simulink model "Fig_9_10__"  (R2024a)
settings: Solver=VariableStepAuto  StartTime=0.0  StopTime=1  RelTol=1e-3
libraries: spsSeriesRLCBranchLib x8, spsThreePhaseVIMeasurementLib x4, spsVoltageMeasurementLib x3, slpidlib x3, spsUniversalBridgeLib x2, spsDiodeLib x2, spsIGBTDiodeLib x2, spsPWMGeneratorDCDCLib x2, spsabctodq0Lib x2, spsCurrentMeasurementLib x2, spsThreePhaseSeriesRLCBranchLib x2, spsThreePhaseSeriesRLCLoadLib x2
settings Model: Creator=MS  LastModifiedBy=Dileep Uppara

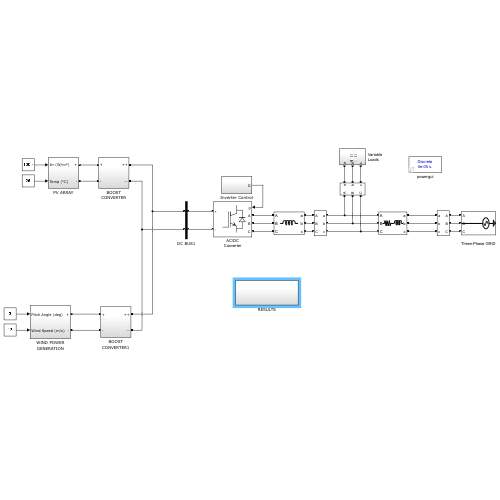
[thumbnail: Simulink's stored preview of the top-level diagram]
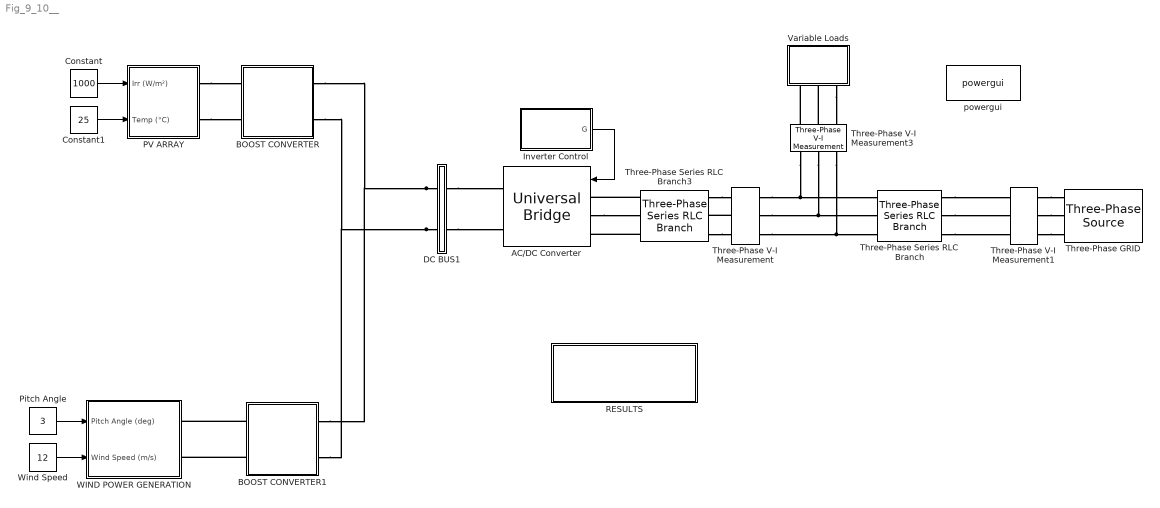
== system Fig_9_10__ ==
  " Three-Phase GRID" : spsThreePhaseSourceLib/Three-Phase Source  InternalConnection=Yg  VoltagePhases=off  Voltage=400  PhaseAngle=0  Voltage_phases=[25e3 25e3 25e3]/sqrt(3)  PhaseAngles_phases=[0 -120 +120]  Frequency=50  NonIdealSource=on  SpecifyImpedance=off  Resistance=0  Inductance=0  ShortCircuitLevel=100e6  BaseVoltage=0  XRratio=7  BusType=swing  Pref=0  Qref=0  Prefabc=[10e3, 10e3, 10e3]  Qrefabc=[0, 0, 0]  Qmin=-inf  Qmax=inf
  AC/DC Converter : spsUniversalBridgeLib/Universal Bridge  Arms=3  SnubberResistance=1e5  SnubberCapacitance=inf  Device=IGBT / Diodes  Ron=1e-3  Lon=0  ForwardVoltages="[  0  0  ]"  ForwardVoltage=0  GTOparameters=[ 10e-6 , 20e-6 ]  IGBTparameters=[ 1e-6 , 2e-6 ]  Measurements=None  Measurements_2=None  converterType=Rectifier
  BOOST CONVERTER : Subsystem
  BOOST CONVERTER1 : Subsystem
  Constant : Constant  Value=1000  SampleTime=50e-6
  Constant1 : Constant  Value=25  SampleTime=50e-6
  DC BUS1 : Subsystem
  Inverter Control : Subsystem
  PV ARRAY : Subsystem
  "Pitch Angle " : Constant  Value=3  SampleTime=50e-6
  RESULTS : Subsystem
  Three-Phase Series RLC Branch : spsThreePhaseSeriesRLCBranchLib/Three-Phase Series RLC Branch  LConnTagsString=A|B|C  RConnTagsString=A|B|C  BranchType=RL  Resistance=2.088  Inductance=0.01e-3  Capacitance=1e-6  Measurements=None
  Three-Phase Series RLC Branch3 : spsThreePhaseSeriesRLCBranchLib/Three-Phase Series RLC Branch  LConnTagsString=A|B|C  RConnTagsString=A|B|C  BranchType=L  Resistance=3  Inductance=20e-3  Capacitance=1e-6  Measurements=None
  Three-Phase V-I Measurement : spsThreePhaseVIMeasurementLib/Three-Phase V-I Measurement  VoltageMeasurement=phase-to-ground  SetLabelV=on  LabelV=Viabc  Vpu=off  VpuLL=off  CurrentMeasurement=yes  SetLabelI=on  LabelI=Iiabc  Ipu=off  Pbase=100e6  Vbase=500e3  OutputType=Complex  PhasorSimulation=off  PSBequivalent=0
  Three-Phase V-I Measurement1 : spsThreePhaseVIMeasurementLib/Three-Phase V-I Measurement  VoltageMeasurement=phase-to-ground  SetLabelV=on  LabelV=Vgabc  Vpu=off  VpuLL=off  CurrentMeasurement=yes  SetLabelI=on  LabelI=Igabc  Ipu=off  Pbase=100e6  Vbase=500e3  OutputType=Complex  PhasorSimulation=off  PSBequivalent=0
  Three-Phase V-I Measurement3 : spsThreePhaseVIMeasurementLib/Three-Phase V-I Measurement  VoltageMeasurement=phase-to-ground  SetLabelV=on  LabelV=Vlabc  Vpu=off  VpuLL=off  CurrentMeasurement=yes  SetLabelI=on  LabelI=Ilabc  Ipu=off  Pbase=100e6  Vbase=500e3  OutputType=Complex  PhasorSimulation=off  PSBequivalent=0
  Variable Loads : Subsystem
  WIND POWER GENERATION : Subsystem
  Wind Speed : Constant  Value=12  SampleTime=50e-6
  powergui : sps_lib/powergui  Priority=1  SimulationMode=Discrete  SampleTime=50e-6  frequency=60  Iterations=50  frequencyindice=0  Pbase=100e6  ErrMax=1e-4  UnitsV=kV  UnitsW=MW  buscounter=0  FunctionMessages=off  echomessages=off  EnableUseOfTLC=off  CurrentSourceSwitches=off  DisableSnubberDevices=off  DisableRonSwitches=off  DisableVfSwitches=off  DisplayEquations=off  AutomaticDiscreteSolvers=off  SolverType=Tustin/Backward Euler (TBE)  Interpol=off  ExternalGateDelay=off  methode=off  Ts=100  x0status=blocks  SPID=on  SwTol=0  HookPort=off  NonlinearTolerance=1e-4  nMaxIteration=100  ContinueOnMaxIteration=off  RestoreLinks=warning  ResistiveCurrentMeasurement=off  Frange=[0:2:500]  Ylog=off  Xlog=on  ShowGrid=off  save=off  variable=ZData  structure=0  ZoomFFT=off  StartTime=0.0  cycles=1  DisplayStyle=1  fundamental=60  FreqAxis=off  MaxFrequency=1000  frequencyindicesteady=1  RmsSteady=1  display=off
  wires:
  Inverter Control/1(G) -> AC/DC Converter/1
  Constant/1 -> PV ARRAY/1(Irr (W/m²))
  Constant1/1 -> PV ARRAY/2(Temp (°C))
  Wind Speed/1 -> WIND POWER GENERATION/2(Wind Speed (m/s))
  "Pitch Angle "/1 -> WIND POWER GENERATION/1(Pitch Angle (deg))
  connections:
  Three-Phase Series RLC Branch3/LConn1 -- AC/DC Converter/LConn1
  AC/DC Converter/LConn2 -- Three-Phase Series RLC Branch3/LConn2
  Three-Phase Series RLC Branch3/LConn3 -- AC/DC Converter/LConn3
  Three-Phase Series RLC Branch3/RConn1 -- Three-Phase V-I Measurement/LConn1
  Three-Phase V-I Measurement/LConn2 -- Three-Phase Series RLC Branch3/RConn2
  Three-Phase Series RLC Branch3/RConn3 -- Three-Phase V-I Measurement/LConn3
  DC BUS1/RConn2 -- AC/DC Converter/RConn2
  DC BUS1/RConn1 -- AC/DC Converter/RConn1
  Three-Phase V-I Measurement3/LConn1 -- Three-Phase Series RLC Branch/LConn1 -- Three-Phase V-I Measurement/RConn1
  Three-Phase V-I Measurement3/LConn3 -- Three-Phase Series RLC Branch/LConn3 -- Three-Phase V-I Measurement/RConn3
  Three-Phase V-I Measurement3/LConn2 -- Three-Phase V-I Measurement/RConn2 -- Three-Phase Series RLC Branch/LConn2
  Three-Phase V-I Measurement1/LConn3 -- " Three-Phase GRID"/RConn3
  Three-Phase Series RLC Branch/RConn1 -- Three-Phase V-I Measurement1/RConn1
  Three-Phase V-I Measurement1/LConn1 -- " Three-Phase GRID"/RConn1
  Three-Phase Series RLC Branch/RConn2 -- Three-Phase V-I Measurement1/RConn2
  Three-Phase V-I Measurement1/LConn2 -- " Three-Phase GRID"/RConn2
  Three-Phase Series RLC Branch/RConn3 -- Three-Phase V-I Measurement1/RConn3
  DC BUS1/LConn2 -- BOOST CONVERTER1/RConn2 -- BOOST CONVERTER/RConn2
  DC BUS1/LConn1 -- BOOST CONVERTER1/RConn1 -- BOOST CONVERTER/RConn1
  Three-Phase V-I Measurement3/RConn2 -- Variable Loads/LConn2
  Three-Phase V-I Measurement3/RConn1 -- Variable Loads/LConn1
  Variable Loads/LConn3 -- Three-Phase V-I Measurement3/RConn3
  PV ARRAY/RConn1 -- BOOST CONVERTER/LConn1
  BOOST CONVERTER1/LConn1 -- WIND POWER GENERATION/RConn1
  BOOST CONVERTER1/LConn2 -- WIND POWER GENERATION/RConn2
  PV ARRAY/RConn2 -- BOOST CONVERTER/LConn2

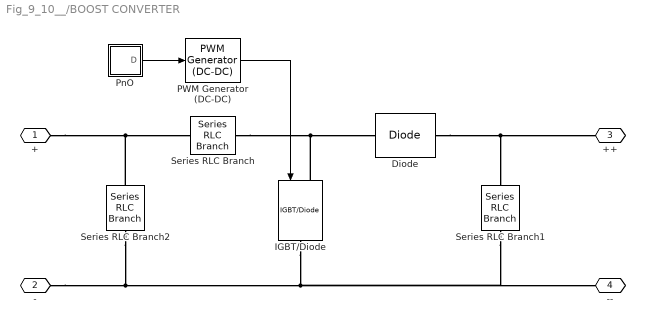
== system Fig_9_10__/BOOST CONVERTER ==
  Diode : spsDiodeLib/Diode  Ron=0.001  Lon=0  Vf=0.8  IC=0  UseSnubber=0  Rs=500  Cs=250e-9  Measurements=off
  IGBT/Diode : spsIGBTDiodeLib/IGBT//Diode  Ron=1e-3  Rs=1e5  Cs=inf  Measurements=off
  PWM Generator (DC-DC) : spsPWMGeneratorDCDCLib/PWM Generator (DC-DC)  Fsw=15e3  Ts=50e-6
  PnO : Subsystem
  Series RLC Branch : spsSeriesRLCBranchLib/Series RLC Branch  LConnTagsString=__new0  RConnTagsString=__new0  BranchType=L  Resistance=0.01  Inductance=0.009e-3  SetiL0=off  InitialCurrent=0  Capacitance=1e-6  Setx0=off  InitialVoltage=0  Measurements=None
  Series RLC Branch1 : spsSeriesRLCBranchLib/Series RLC Branch  LConnTagsString=__new0  RConnTagsString=__new0  BranchType=C  Resistance=0.01  Inductance=0.5e-3  SetiL0=off  InitialCurrent=0  Capacitance=880e-6  Setx0=off  InitialVoltage=0  Measurements=None
  Series RLC Branch2 : spsSeriesRLCBranchLib/Series RLC Branch  LConnTagsString=__new0  RConnTagsString=__new0  BranchType=C  Resistance=0.01  Inductance=0.5e-3  SetiL0=off  InitialCurrent=0  Capacitance=880e-6  Setx0=off  InitialVoltage=0  Measurements=None
  + : PMIOPort  Side=Left
  - : PMIOPort  Port=2  Side=Left
  ++ : PMIOPort  Port=3  Side=Right
  -- : PMIOPort  Port=4  Side=Right
  wires:
  PWM Generator (DC-DC)/1 -> IGBT/Diode/1
  PnO/1(D) -> PWM Generator (DC-DC)/1
  connections:
  Series RLC Branch/RConn1 -- Diode/LConn1 -- IGBT/Diode/LConn1
  +/RConn1 -- Series RLC Branch2/LConn1 -- Series RLC Branch/LConn1
  Series RLC Branch2/RConn1 -- -/RConn1 -- Series RLC Branch1/RConn1 -- --/RConn1 -- IGBT/Diode/RConn1
  Diode/RConn1 -- ++/RConn1 -- Series RLC Branch1/LConn1

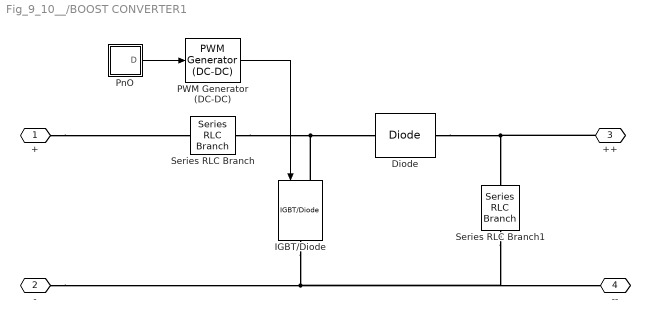
== system Fig_9_10__/BOOST CONVERTER1 ==
  Diode : spsDiodeLib/Diode  Ron=0.001  Lon=0  Vf=0.8  IC=0  UseSnubber=0  Rs=500  Cs=250e-9  Measurements=off
  IGBT/Diode : spsIGBTDiodeLib/IGBT//Diode  Ron=1e-3  Rs=1e5  Cs=inf  Measurements=off
  PWM Generator (DC-DC) : spsPWMGeneratorDCDCLib/PWM Generator (DC-DC)  Fsw=15e3  Ts=50e-6
  PnO : Subsystem
  Series RLC Branch : spsSeriesRLCBranchLib/Series RLC Branch  LConnTagsString=__new0  RConnTagsString=__new0  BranchType=RL  Resistance=1.524  Inductance=0.1e-3  SetiL0=off  InitialCurrent=0  Capacitance=1e-6  Setx0=off  InitialVoltage=0  Measurements=None
  Series RLC Branch1 : spsSeriesRLCBranchLib/Series RLC Branch  LConnTagsString=__new0  RConnTagsString=__new0  BranchType=C  Resistance=0.01  Inductance=0.5e-3  SetiL0=off  InitialCurrent=0  Capacitance=880e-6  Setx0=off  InitialVoltage=0  Measurements=None
  + : PMIOPort  Side=Left
  - : PMIOPort  Port=2  Side=Left
  ++ : PMIOPort  Port=3  Side=Right
  -- : PMIOPort  Port=4  Side=Right
  wires:
  PWM Generator (DC-DC)/1 -> IGBT/Diode/1
  PnO/1(D) -> PWM Generator (DC-DC)/1
  connections:
  Series RLC Branch/RConn1 -- Diode/LConn1 -- IGBT/Diode/LConn1
  Diode/RConn1 -- Series RLC Branch1/LConn1 -- ++/RConn1
  +/RConn1 -- Series RLC Branch/LConn1
  -/RConn1 -- Series RLC Branch1/RConn1 -- --/RConn1 -- IGBT/Diode/RConn1

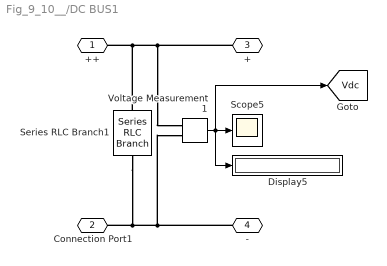
== system Fig_9_10__/DC BUS1 ==
  Display5 : Display
  Scope5 : Scope
  Series RLC Branch1 : spsSeriesRLCBranchLib/Series RLC Branch  LConnTagsString=__new0  RConnTagsString=__new0  BranchType=C  Resistance=0.01  Inductance=0.5e-3  SetiL0=off  InitialCurrent=0  Capacitance=10000e-6  Setx0=off  InitialVoltage=0  Measurements=None
  Voltage Measurement1 : spsVoltageMeasurementLib/Voltage Measurement  PhasorSimulation=off  OutputType=Complex  PSBequivalent=0
  ++ : PMIOPort  Side=Left
  Connection Port1 : PMIOPort  Port=2  Side=Left
  + : PMIOPort  Port=3  Side=Right
  - : PMIOPort  Port=4  Side=Right
  tag scope: Vdc=global
  wires:
  Voltage Measurement1/1 -> [Vdc], Display5/1, Scope5/1
  connections:
  -/RConn1 -- Voltage Measurement1/LConn2 -- Series RLC Branch1/RConn1 -- Connection Port1/RConn1
  +/RConn1 -- Series RLC Branch1/LConn1 -- ++/RConn1 -- Voltage Measurement1/LConn1

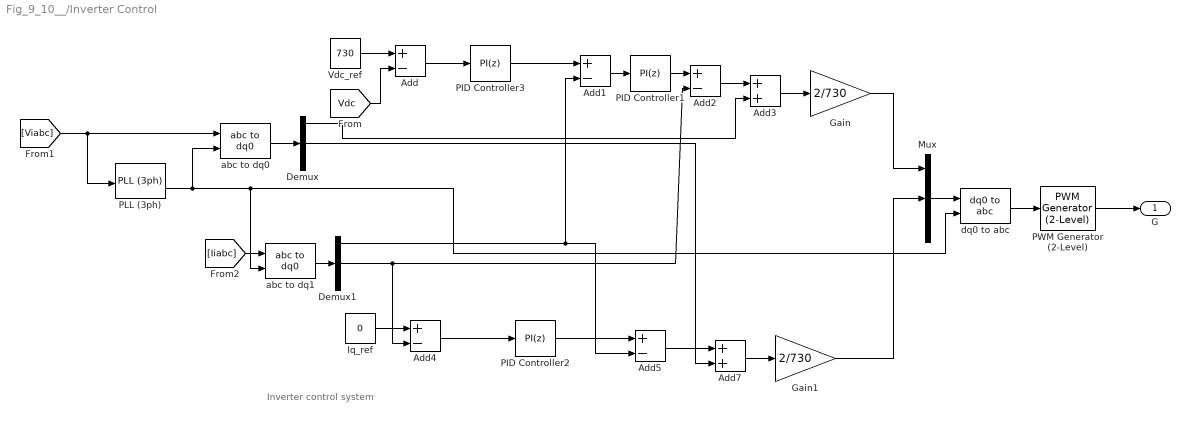
== system Fig_9_10__/Inverter Control ==
  note: Inverter control system
  Add{,1..2,4..5} (5 alike) : Sum  Inputs=+-
  Add3 : Sum
  Add7 : Sum
  Demux : Demux  Outputs=3
  Demux1 : Demux  Outputs=3
  Gain : Gain  Gain=2/730
  Gain1 : Gain  Gain=2/730
  Iq_ref : Constant  Value=0
  Mux : Mux  Inputs=3
  PID Controller1 : slpidlib/PID Controller  Controller=PI  Form=Parallel  TimeDomain=Discrete-time  UseExternalTs=off  SampleTime=-1  IntegratorMethod=Forward Euler  FilterMethod=Forward Euler  ControllerParametersSource=internal  P=0.5  I=200  UseKiTs=off  D=0  UseExternalDerivativeSource=off  N=100  UseFilter=on  TunerSelectOption=Transfer Function Based (PID Tuner App)  InitialConditionSource=internal  InitialConditionForIntegrator=0  InitialConditionForFilter=0  DifferentiatorICPrevScaledInput=0  ExternalReset=none  TrackingMode=off  Kt=1  LimitOutput=off  SatLimitsSource=internal  UpperSaturationLimit=inf  LowerSaturationLimit=-inf  LinearizeAsGain=on  AntiWindupMode=none  Kb=1  LimitIntegrator=off  UpperIntegratorSaturationLimit=inf  LowerIntegratorSaturationLimit=-inf  POutMin=[]  POutMax=[]  IOutMin=[]  IOutMax=[]  DOutMin=[]  DOutMax=[]  NOutMin=[]  NOutMax=[]  SumOutMin=[]  SumOutMax=[]  SaturationOutMin=[]  SaturationOutMax=[]  PParamMin=[]  PParamMax=[]  IParamMin=[]  IParamMax=[]  DParamMin=[]  DParamMax=[]  NParamMin=[]  NParamMax=[]  KbParamMin=[]  KbParamMax=[]  KtParamMin=[]  KtParamMax=[]  KbOutMin=[]  KbOutMax=[]  KtOutMin=[]  KtOutMax=[]  IntegratorOutMin=[]  IntegratorOutMax=[]  FilterOutMin=[]  FilterOutMax=[]  SumI1OutMin=[]  SumI1OutMax=[]  SumI2OutMin=[]  SumI2OutMax=[]  SumI3OutMin=[]  SumI3OutMax=[]  SumI4OutMin=[]  SumI4OutMax=[]  SumDOutMin=[]  SumDOutMax=[]  DifferentiatorOutMin=[]  DifferentiatorOutMax=[]  FilterDiffOutCoefMin=[]  FilterDiffOutCoefMax=[]  ReciprocalOutMin=[]  ReciprocalOutMax=[]  SumDenOutMin=[]  SumDenOutMax=[]  SumNumOutMin=[]  SumNumOutMax=[]  DivideOutMin=[]  DivideOutMax=[]  UdiffTsProdOutMin=[]  UdiffTsProdOutMax=[]  NTsProdOutMin=[]  NTsProdOutMax=[]  UintegralTsProdOutMin=[]  UintegralTsProdOutMax=[]  UngainTsProdOutMin=[]  UngainTsProdOutMax=[]  ClampingZeroOutDataTypeStr=Inherit: Inherit via back propagation  ClampingZeroOutMin=[]  ClampingZeroOutMax=[]  FilterDenConstantOutDataTypeStr=Inherit: Inherit via back propagation  FilterDenConstantOutMin=[]  FilterDenConstantOutMax=[]  PCopyOutDataTypeStr=Inherit: Inherit via back propagation  PCopyOutMin=[]  PCopyOutMax=[]  NCopyOutDataTypeStr=Inherit: Inherit via back propagation  NCopyOutMin=[]  NCopyOutMax=[]  IntegratorContinuousStateAttributes=''  IntegratorStateMustResolveToSignalObject=off  IntegratorRTWStateStorageClass=Auto  FilterContinuousStateAttributes=''  FilterStateMustResolveToSignalObject=off  FilterRTWStateStorageClass=Auto  ParallelPVariant=InternalParameters  IdealPVariant=Disabled  IVariant=InternalParameters  DVariant=Disabled  IntegratorVariant=Discrete  SatVariant=Disabled  AWVariant=Passthrough  PCopyVariant=Disabled  TRVariant=Disabled  FdbkBlocksVariant=Forward  IdealPFdbkVariant=Disabled  SatFdbkVariant=Disabled  DerivativeFilterVariant=Disabled  NVariant=Disabled  NCopyVariant=Disabled_SignalSpec  FilterICVariant=Disabled  IntegratorICVariant=InternalICs  ExternalResetVariant=Disabled  TRSumVariant=Passthrough  SumFdbkVariant=Disabled  SumVariant=Sum_PI  TsampFilterVariant=InternalTs  TsampNgainVariant=Passthrough  TsampIntegralVariant=Disabled_SignalSpec  ExternalSaturationOutDataTypeStr=Inherit: Same as second input  DerivativeSourceVariant=Disabled
  PID Controller2 : slpidlib/PID Controller  Controller=PI  Form=Parallel  TimeDomain=Discrete-time  UseExternalTs=off  SampleTime=-1  IntegratorMethod=Forward Euler  FilterMethod=Forward Euler  ControllerParametersSource=internal  P=0.5  I=200  UseKiTs=off  D=0  UseExternalDerivativeSource=off  N=100  UseFilter=on  TunerSelectOption=Transfer Function Based (PID Tuner App)  InitialConditionSource=internal  InitialConditionForIntegrator=0  InitialConditionForFilter=0  DifferentiatorICPrevScaledInput=0  ExternalReset=none  TrackingMode=off  Kt=1  LimitOutput=off  SatLimitsSource=internal  UpperSaturationLimit=inf  LowerSaturationLimit=-inf  LinearizeAsGain=on  AntiWindupMode=none  Kb=1  LimitIntegrator=off  UpperIntegratorSaturationLimit=inf  LowerIntegratorSaturationLimit=-inf  POutMin=[]  POutMax=[]  IOutMin=[]  IOutMax=[]  DOutMin=[]  DOutMax=[]  NOutMin=[]  NOutMax=[]  SumOutMin=[]  SumOutMax=[]  SaturationOutMin=[]  SaturationOutMax=[]  PParamMin=[]  PParamMax=[]  IParamMin=[]  IParamMax=[]  DParamMin=[]  DParamMax=[]  NParamMin=[]  NParamMax=[]  KbParamMin=[]  KbParamMax=[]  KtParamMin=[]  KtParamMax=[]  KbOutMin=[]  KbOutMax=[]  KtOutMin=[]  KtOutMax=[]  IntegratorOutMin=[]  IntegratorOutMax=[]  FilterOutMin=[]  FilterOutMax=[]  SumI1OutMin=[]  SumI1OutMax=[]  SumI2OutMin=[]  SumI2OutMax=[]  SumI3OutMin=[]  SumI3OutMax=[]  SumI4OutMin=[]  SumI4OutMax=[]  SumDOutMin=[]  SumDOutMax=[]  DifferentiatorOutMin=[]  DifferentiatorOutMax=[]  FilterDiffOutCoefMin=[]  FilterDiffOutCoefMax=[]  ReciprocalOutMin=[]  ReciprocalOutMax=[]  SumDenOutMin=[]  SumDenOutMax=[]  SumNumOutMin=[]  SumNumOutMax=[]  DivideOutMin=[]  DivideOutMax=[]  UdiffTsProdOutMin=[]  UdiffTsProdOutMax=[]  NTsProdOutMin=[]  NTsProdOutMax=[]  UintegralTsProdOutMin=[]  UintegralTsProdOutMax=[]  UngainTsProdOutMin=[]  UngainTsProdOutMax=[]  ClampingZeroOutDataTypeStr=Inherit: Inherit via back propagation  ClampingZeroOutMin=[]  ClampingZeroOutMax=[]  FilterDenConstantOutDataTypeStr=Inherit: Inherit via back propagation  FilterDenConstantOutMin=[]  FilterDenConstantOutMax=[]  PCopyOutDataTypeStr=Inherit: Inherit via back propagation  PCopyOutMin=[]  PCopyOutMax=[]  NCopyOutDataTypeStr=Inherit: Inherit via back propagation  NCopyOutMin=[]  NCopyOutMax=[]  IntegratorContinuousStateAttributes=''  IntegratorStateMustResolveToSignalObject=off  IntegratorRTWStateStorageClass=Auto  FilterContinuousStateAttributes=''  FilterStateMustResolveToSignalObject=off  FilterRTWStateStorageClass=Auto  ParallelPVariant=InternalParameters  IdealPVariant=Disabled  IVariant=InternalParameters  DVariant=Disabled  IntegratorVariant=Discrete  SatVariant=Disabled  AWVariant=Passthrough  PCopyVariant=Disabled  TRVariant=Disabled  FdbkBlocksVariant=Forward  IdealPFdbkVariant=Disabled  SatFdbkVariant=Disabled  DerivativeFilterVariant=Disabled  NVariant=Disabled  NCopyVariant=Disabled_SignalSpec  FilterICVariant=Disabled  IntegratorICVariant=InternalICs  ExternalResetVariant=Disabled  TRSumVariant=Passthrough  SumFdbkVariant=Disabled  SumVariant=Sum_PI  TsampFilterVariant=InternalTs  TsampNgainVariant=Passthrough  TsampIntegralVariant=Disabled_SignalSpec  ExternalSaturationOutDataTypeStr=Inherit: Same as second input  DerivativeSourceVariant=Disabled
  PID Controller3 : slpidlib/PID Controller  Controller=PI  Form=Parallel  TimeDomain=Discrete-time  UseExternalTs=off  SampleTime=-1  IntegratorMethod=Forward Euler  FilterMethod=Forward Euler  ControllerParametersSource=internal  P=1  I=500  UseKiTs=off  D=0  UseExternalDerivativeSource=off  N=100  UseFilter=on  TunerSelectOption=Transfer Function Based (PID Tuner App)  InitialConditionSource=internal  InitialConditionForIntegrator=0  InitialConditionForFilter=0  DifferentiatorICPrevScaledInput=0  ExternalReset=none  TrackingMode=off  Kt=1  LimitOutput=off  SatLimitsSource=internal  UpperSaturationLimit=inf  LowerSaturationLimit=-inf  LinearizeAsGain=on  AntiWindupMode=none  Kb=1  LimitIntegrator=off  UpperIntegratorSaturationLimit=inf  LowerIntegratorSaturationLimit=-inf  POutMin=[]  POutMax=[]  IOutMin=[]  IOutMax=[]  DOutMin=[]  DOutMax=[]  NOutMin=[]  NOutMax=[]  SumOutMin=[]  SumOutMax=[]  SaturationOutMin=[]  SaturationOutMax=[]  PParamMin=[]  PParamMax=[]  IParamMin=[]  IParamMax=[]  DParamMin=[]  DParamMax=[]  NParamMin=[]  NParamMax=[]  KbParamMin=[]  KbParamMax=[]  KtParamMin=[]  KtParamMax=[]  KbOutMin=[]  KbOutMax=[]  KtOutMin=[]  KtOutMax=[]  IntegratorOutMin=[]  IntegratorOutMax=[]  FilterOutMin=[]  FilterOutMax=[]  SumI1OutMin=[]  SumI1OutMax=[]  SumI2OutMin=[]  SumI2OutMax=[]  SumI3OutMin=[]  SumI3OutMax=[]  SumI4OutMin=[]  SumI4OutMax=[]  SumDOutMin=[]  SumDOutMax=[]  DifferentiatorOutMin=[]  DifferentiatorOutMax=[]  FilterDiffOutCoefMin=[]  FilterDiffOutCoefMax=[]  ReciprocalOutMin=[]  ReciprocalOutMax=[]  SumDenOutMin=[]  SumDenOutMax=[]  SumNumOutMin=[]  SumNumOutMax=[]  DivideOutMin=[]  DivideOutMax=[]  UdiffTsProdOutMin=[]  UdiffTsProdOutMax=[]  NTsProdOutMin=[]  NTsProdOutMax=[]  UintegralTsProdOutMin=[]  UintegralTsProdOutMax=[]  UngainTsProdOutMin=[]  UngainTsProdOutMax=[]  ClampingZeroOutDataTypeStr=Inherit: Inherit via back propagation  ClampingZeroOutMin=[]  ClampingZeroOutMax=[]  FilterDenConstantOutDataTypeStr=Inherit: Inherit via back propagation  FilterDenConstantOutMin=[]  FilterDenConstantOutMax=[]  PCopyOutDataTypeStr=Inherit: Inherit via back propagation  PCopyOutMin=[]  PCopyOutMax=[]  NCopyOutDataTypeStr=Inherit: Inherit via back propagation  NCopyOutMin=[]  NCopyOutMax=[]  IntegratorContinuousStateAttributes=''  IntegratorStateMustResolveToSignalObject=off  IntegratorRTWStateStorageClass=Auto  FilterContinuousStateAttributes=''  FilterStateMustResolveToSignalObject=off  FilterRTWStateStorageClass=Auto  ParallelPVariant=InternalParameters  IdealPVariant=Disabled  IVariant=InternalParameters  DVariant=Disabled  IntegratorVariant=Discrete  SatVariant=Disabled  AWVariant=Passthrough  PCopyVariant=Disabled  TRVariant=Disabled  FdbkBlocksVariant=Forward  IdealPFdbkVariant=Disabled  SatFdbkVariant=Disabled  DerivativeFilterVariant=Disabled  NVariant=Disabled  NCopyVariant=Disabled_SignalSpec  FilterICVariant=Disabled  IntegratorICVariant=InternalICs  ExternalResetVariant=Disabled  TRSumVariant=Passthrough  SumFdbkVariant=Disabled  SumVariant=Sum_PI  TsampFilterVariant=InternalTs  TsampNgainVariant=Passthrough  TsampIntegralVariant=Disabled_SignalSpec  ExternalSaturationOutDataTypeStr=Inherit: Same as second input  DerivativeSourceVariant=Disabled
  PLL (3ph) : spsPLL3phLib/PLL (3ph)  Fmin=45  Par_Init=[0, 50]  ParK=[180, 3200, 1]  TcD=1e-4  MaxRateChangeFreq=12  FilterCutOffFreq=25  Ts=50e-6  AGC=on
  PWM Generator (2-Level) : spsPWMGenerator2LevelLib/PWM Generator (2-Level)  ModulatorType=Three-phase bridge (6 pulses)  ModulatorMode=Unsynchronized  Fc=20e3  Pc=90  nF=27  MinMax="[ -1  1 ]"  SamplingTechnique=Natural  ModulatingSignals=off  m=0.8  Freq=50  Phase=0  Ts=50e-6  ShowCarrierOutport=off
  Vdc_ref : Constant  Value=730
  abc to dq0 : spsabctodq0Lib/abc to dq0  Alignment=90 degrees behind phase A axis
  abc to dq1 : spsabctodq0Lib/abc to dq0  Alignment=90 degrees behind phase A axis
  dq0 to abc : spsdq0toabcLib/dq0 to abc  Alignment=90 degrees behind phase A axis
  G : Outport
  wires:
  Vdc_ref/1 -> Add/1
  [Vdc] -> Add/2
  Add1/1 -> PID Controller1/1
  PID Controller1/1 -> Add2/1
  Add2/1 -> Add3/1
  Add3/1 -> Gain/1
  abc to dq0/1 -> Demux/1
  [Viabc] -> PLL (3ph)/1, abc to dq0/1
  PLL (3ph)/2 -> dq0 to abc/2, abc to dq1/2, abc to dq0/2
  [Iiabc] -> abc to dq1/1
  abc to dq1/1 -> Demux1/1
  Add5/1 -> Add7/1
  PID Controller2/1 -> Add5/1
  Add4/1 -> PID Controller2/1
  Demux1/2 -> Add4/2, Add2/2
  Iq_ref/1 -> Add4/1
  Demux/1 -> Add3/2
  Demux1/1 -> Add5/2, Add1/2
  Add7/1 -> Gain1/1
  Demux/2 -> Add7/2
  Gain/1 -> Mux/1
  Mux/1 -> dq0 to abc/1
  Gain1/1 -> Mux/2
  dq0 to abc/1 -> PWM Generator (2-Level)/1
  PWM Generator (2-Level)/1 -> G/1
  PID Controller3/1 -> Add1/1
  Add/1 -> PID Controller3/1

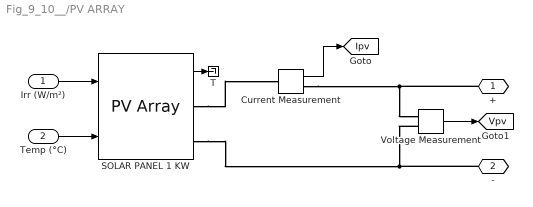
== system Fig_9_10__/PV ARRAY ==
  Irr (W/m²) : Inport
  Temp (°C) : Inport  Port=2
  Current Measurement : spsCurrentMeasurementLib/Current Measurement  PhasorSimulation=off  OutputType=Complex  PSBequivalent=0
  SOLAR PANEL 1 KW : spsPVArrayLib/PV Array  Npar=44  Nser=18  PlotType=array @ 1000 W/m2 & specified temperatures  S_vec="[ 1000  500  100 ]"  Temp_C_vec="[ 45 25  ]"  ModuleName=User-defined  PlotWhenSelected=off  Pm=214.6493  Ncell=60  Voc=36.3  Isc=7.84  Vm=29  Im=7.4017  beta_Voc_pc=-0.36099  alpha_Isc_pc=0.102  beta_Voc=-0.13104  alpha_Isc=0.0079968  IL=7.9095  I0=2.9374e-10  nI=0.98114  Rsh=294.0158  Rs=0.39142  RobustModel=off  RobustCellTemperature=313.3991  BAL=on  Tc=1e-6  Tfilter=5e-5
  T : Terminator
  Voltage Measurement : spsVoltageMeasurementLib/Voltage Measurement  PhasorSimulation=off  OutputType=Complex  PSBequivalent=0
  + : PMIOPort  Side=Right
  - : PMIOPort  Port=2  Side=Right
  tag scope: Ipv=global, Vpv=global
  wires:
  Voltage Measurement/1 -> [Vpv]
  Current Measurement/1 -> [Ipv]
  SOLAR PANEL 1 KW/1 -> T/1
  Irr (W/m²)/1 -> SOLAR PANEL 1 KW/1
  Temp (°C)/1 -> SOLAR PANEL 1 KW/2
  connections:
  Current Measurement/RConn1 -- +/RConn1 -- Voltage Measurement/LConn1
  Voltage Measurement/LConn2 -- -/RConn1 -- SOLAR PANEL 1 KW/RConn2
  SOLAR PANEL 1 KW/RConn1 -- Current Measurement/LConn1

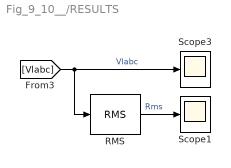
== system Fig_9_10__/RESULTS ==
  RMS : spsRMSLib/RMS  TrueRMS=on  Freq=50  RMSInit=0  Ts=50e-6
  Scope1 : Scope
  Scope3 : Scope
  wires:
  RMS/1 -> Scope1/1  "Rms"
  [Vlabc] -> RMS/1, Scope3/1  "Vlabc"

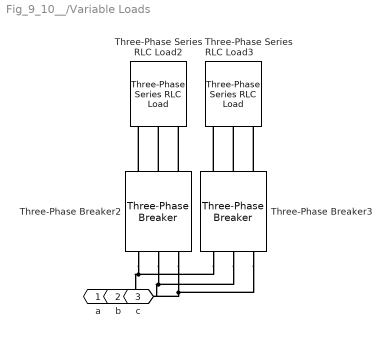
== system Fig_9_10__/Variable Loads ==
  Three-Phase Series RLC Load2 : spsThreePhaseSeriesRLCLoadLib/Three-Phase Series RLC Load  LConnTagsString=A|B|C  Configuration=Y (grounded)  NominalVoltage=400  Vabc=[1e3 1e3 1e3]  Vabcp=[1e3 1e3 1e3]  NominalFrequency=50  UnbalancedPower=off  ActivePower=20e3  InductivePower=0  CapacitivePower=0  Pabc=[10e3 9e3 11e3]  QLabc=[100 90 110]  QCabc=[100 90 110]  Pabcp=[10e3 9e3 11e3]  QLabcp=[100 90 110]  QCabcp=[100 90 110]  Measurements=None  LoadType=constant Z
  Three-Phase Series RLC Load3 : spsThreePhaseSeriesRLCLoadLib/Three-Phase Series RLC Load  LConnTagsString=A|B|C  Configuration=Y (grounded)  NominalVoltage=400  Vabc=[1e3 1e3 1e3]  Vabcp=[1e3 1e3 1e3]  NominalFrequency=50  UnbalancedPower=off  ActivePower=20e3  InductivePower=0  CapacitivePower=0  Pabc=[10e3 9e3 11e3]  QLabc=[100 90 110]  QCabc=[100 90 110]  Pabcp=[10e3 9e3 11e3]  QLabcp=[100 90 110]  QCabcp=[100 90 110]  Measurements=None  LoadType=constant Z
  Three-Phase Breaker2 : spsThreePhaseBreakerLib/Three-Phase Breaker  InitialState=open  SwitchA=on  SwitchB=on  SwitchC=on  SwitchTimes=[0.2 0.4]  External=off  BreakerResistance=0.01  SnubberResistance=1e6  SnubberCapacitance=inf  Measurements=None
  Three-Phase Breaker3 : spsThreePhaseBreakerLib/Three-Phase Breaker  InitialState=closed  SwitchA=on  SwitchB=on  SwitchC=on  SwitchTimes=[0.6 0.8]  External=off  BreakerResistance=0.01  SnubberResistance=1e6  SnubberCapacitance=inf  Measurements=None
  a : PMIOPort  Side=Left
  b : PMIOPort  Port=2  Side=Left
  c : PMIOPort  Port=3  Side=Left
  connections:
  Three-Phase Breaker2/LConn3 -- Three-Phase Series RLC Load2/LConn3
  Three-Phase Breaker3/LConn3 -- Three-Phase Series RLC Load3/LConn3
  Three-Phase Breaker2/RConn3 -- c/RConn1 -- Three-Phase Breaker3/RConn3
  Three-Phase Breaker2/RConn2 -- b/RConn1 -- Three-Phase Breaker3/RConn2
  Three-Phase Breaker3/LConn2 -- Three-Phase Series RLC Load3/LConn2
  Three-Phase Breaker2/RConn1 -- a/RConn1 -- Three-Phase Breaker3/RConn1
  Three-Phase Breaker2/LConn2 -- Three-Phase Series RLC Load2/LConn2
  Three-Phase Breaker3/LConn1 -- Three-Phase Series RLC Load3/LConn1
  Three-Phase Breaker2/LConn1 -- Three-Phase Series RLC Load2/LConn1

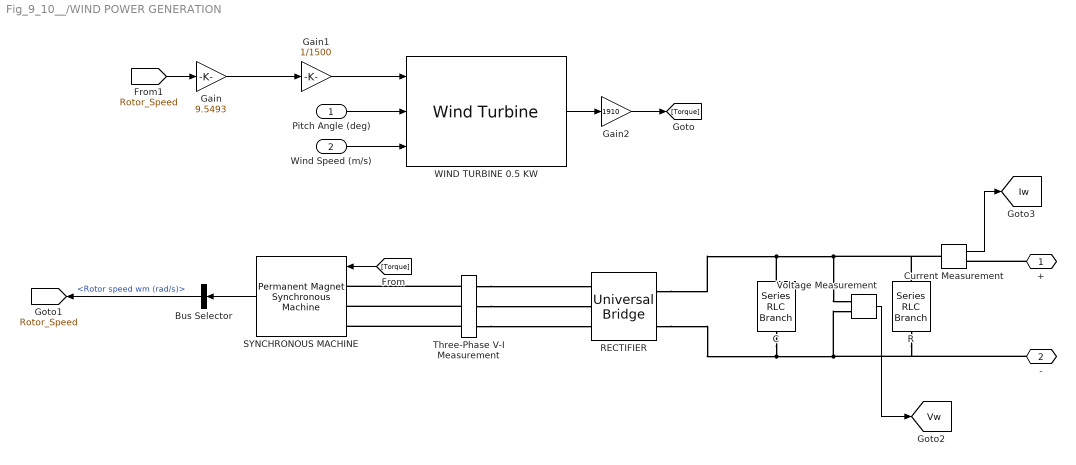
== system Fig_9_10__/WIND POWER GENERATION ==
  Pitch Angle (deg) : Inport
  Wind Speed (m/s) : Inport  Port=2
  Bus Selector : BusSelector  OutputSignals=Rotor speed wm (rad/s)
  C : spsSeriesRLCBranchLib/Series RLC Branch  LConnTagsString=__new0  RConnTagsString=__new0  BranchType=C  Resistance=20  Inductance=1e-3  SetiL0=off  InitialCurrent=0  Capacitance=1000e-6  Setx0=off  InitialVoltage=0  Measurements=None
  Current Measurement : spsCurrentMeasurementLib/Current Measurement  PhasorSimulation=off  OutputType=Complex  PSBequivalent=0
  Gain : Gain  Gain=9.5493
  Gain1 : Gain  Gain=1/1500
  Gain2 : Gain  Gain=1910
  R : spsSeriesRLCBranchLib/Series RLC Branch  LConnTagsString=__new0  RConnTagsString=__new0  BranchType=R  Resistance=15  Inductance=1e-3  SetiL0=off  InitialCurrent=0  Capacitance=10e-3  Setx0=off  InitialVoltage=0  Measurements=None
  RECTIFIER : spsUniversalBridgeLib/Universal Bridge  Arms=3  SnubberResistance=1e5  SnubberCapacitance=inf  Device=Diodes  Ron=1e-3  Lon=0  ForwardVoltages="[  0  0  ]"  ForwardVoltage=0  GTOparameters=[ 10e-6 , 20e-6 ]  IGBTparameters=[ 1e-6 , 2e-6 ]  Measurements=None  Measurements_2=None  converterType=Rectifier
  SYNCHRONOUS MACHINE : spsPermanentMagnetSynchronousMachineLib/Permanent Magnet Synchronous Machine  NbPhases=3  FluxDistribution=Sinusoidal  RotorType=Round  MechanicalLoad=Torque Tm  PresetModel=No  ShowDetailedParameters=on  MeasurementBus=off  Resistance=0.0485  Inductance=8.5e-3  dqInductances=[8.5e-3,8.5e-3]  La=0.000395  MachineConstant=Flux linkage established by magnets (V.s)  Flux=1.2  VoltageCst=870.6237  TorqueCst=7.2  Flat=120  Mechanical=[0.0027 0.0004924 4 0]  PolePairs=4  InitialConditions=[0,0, 0,0]  InitialConditions5ph=[0 0 0 0 0 0]  RefAngle=90 degrees behind phase A axis (modified Park)  IterativeDiscreteModel=Trapezoidal non iterative  TsBlock=50e-6  TsPowergui=0
  Three-Phase V-I Measurement : spsThreePhaseVIMeasurementLib/Three-Phase V-I Measurement  VoltageMeasurement=phase-to-phase  SetLabelV=on  LabelV=Vabc  Vpu=off  VpuLL=off  CurrentMeasurement=yes  SetLabelI=on  LabelI=Iabc  Ipu=off  Pbase=100e6  Vbase=500e3  OutputType=Complex  PhasorSimulation=off  PSBequivalent=0
  Voltage Measurement : spsVoltageMeasurementLib/Voltage Measurement  PhasorSimulation=off  OutputType=Complex  PSBequivalent=0
  WIND TURBINE 0.5 KW : spsWindTurbineLib/Wind Turbine  Pnom=300e3  Pelec_base=300e3/0.9  wind_base=12  P_wind_base=0.73  speed_nom=1.2  pitch_angle=0  c1_c6="[0.51763          116          0.4            5           21     0.006795]"  cp_nom=0.48  lambda_nom=8.1
  + : PMIOPort  Side=Right
  - : PMIOPort  Port=2  Side=Right
  tag scope: Iw=global, Rotor_Speed=global, Vw=global
  wires:
  [Rotor_Speed] -> Gain/1
  WIND TURBINE 0.5 KW/1 -> Gain2/1
  Pitch Angle (deg)/1 -> WIND TURBINE 0.5 KW/2
  Wind Speed (m/s)/1 -> WIND TURBINE 0.5 KW/3
  [Torque] -> SYNCHRONOUS MACHINE/1
  Bus Selector/1 -> [Rotor_Speed]  "<Rotor speed wm (rad/s)>"
  SYNCHRONOUS MACHINE/1 -> Bus Selector/1
  Gain/1 -> Gain1/1
  Gain1/1 -> WIND TURBINE 0.5 KW/1
  Gain2/1 -> [Torque]
  Voltage Measurement/1 -> [Vw]
  Current Measurement/1 -> [Iw]
  connections:
  C/RConn1 -- RECTIFIER/RConn2 -- Voltage Measurement/LConn2 -- -/RConn1 -- R/RConn1
  Three-Phase V-I Measurement/RConn1 -- RECTIFIER/LConn1
  Three-Phase V-I Measurement/LConn2 -- SYNCHRONOUS MACHINE/LConn2
  Three-Phase V-I Measurement/LConn3 -- SYNCHRONOUS MACHINE/LConn3
  Three-Phase V-I Measurement/RConn2 -- RECTIFIER/LConn2
  Three-Phase V-I Measurement/RConn3 -- RECTIFIER/LConn3
  Three-Phase V-I Measurement/LConn1 -- SYNCHRONOUS MACHINE/LConn1
  RECTIFIER/RConn1 -- C/LConn1 -- Voltage Measurement/LConn1 -- Current Measurement/LConn1 -- R/LConn1
  +/RConn1 -- Current Measurement/RConn1

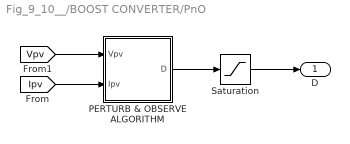
== system Fig_9_10__/BOOST CONVERTER/PnO ==
  PERTURB & OBSERVE ALGORITHM : MATLAB Function  TreatAsAtomicUnit=on
  Saturation : Saturate  UpperLimit=0.2  LowerLimit=0.15
  D : Outport
  wires:
  [Vpv] -> PERTURB & OBSERVE ALGORITHM/1(Vpv)
  [Ipv] -> PERTURB & OBSERVE ALGORITHM/2(Ipv)
  PERTURB & OBSERVE ALGORITHM/1(D) -> Saturation/1
  Saturation/1 -> D/1

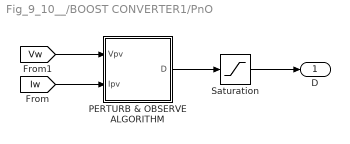
== system Fig_9_10__/BOOST CONVERTER1/PnO ==
  PERTURB & OBSERVE ALGORITHM : MATLAB Function  TreatAsAtomicUnit=on
  Saturation : Saturate  UpperLimit=1  LowerLimit=0
  D : Outport
  wires:
  [Vw] -> PERTURB & OBSERVE ALGORITHM/1(Vpv)
  [Iw] -> PERTURB & OBSERVE ALGORITHM/2(Ipv)
  PERTURB & OBSERVE ALGORITHM/1(D) -> Saturation/1
  Saturation/1 -> D/1

== matlab function Fig_9_10__/BOOST CONVERTER/PnO/PERTURB & OBSERVE ALGORITHM ==
  data: Vpv input; D output; Ipv input
function D = PnO(Vpv, Ipv)

persistent Dprev Pprev Vprev

if isempty(Dprev)
    Dprev = 0.7;
    Vprev = 145;
    Pprev = 1000;
end

deltaD = 125e-6

% Caluclate PV Power
Ppv = Vpv*Ipv

% Increase or decrease duty cycle based on conditions
if (Ppv-Pprev) ~= 0
    if (Ppv-Pprev) > 0
        if (Vpv-Vprev) > 0
            D = Dprev - deltaD;
        else
            D = Dprev + deltaD;
        end
    else
        if (Vpv - Vprev) > 0
            D = Dprev + deltaD;
        else
            D = Dprev - deltaD;
        end
    end
else
    D = Dprev;
end

% Update interval values
Dprev = D;
Vprev = Vpv;
Pprev = Ppv;

== matlab function Fig_9_10__/BOOST CONVERTER1/PnO/PERTURB & OBSERVE ALGORITHM ==
  data: Vpv input; D output; Ipv input
function D = PnO(Vpv, Ipv)

persistent Dprev Pprev Vprev

if isempty(Dprev)
    Dprev = 0.7;
    Vprev = 145;
    Pprev = 1000;
end

deltaD = 125e-6

% Caluclate PV Power
Ppv = Vpv*Ipv

% Increase or decrease duty cycle based on conditions
if (Ppv-Pprev) ~= 0
    if (Ppv-Pprev) > 0
        if (Vpv-Vprev) > 0
            D = Dprev - deltaD;
        else
            D = Dprev + deltaD;
        end
    else
        if (Vpv - Vprev) > 0
            D = Dprev + deltaD;
        else
            D = Dprev - deltaD;
        end
    end
else
    D = Dprev;
end

% Update interval values
Dprev = D;
Vprev = Vpv;
Pprev = Ppv;
